simulink model "dead_time_generator"  (R2023b)
settings: Solver=VariableStepAuto  StartTime=0.0  StopTime=10.0  RelTol=1e-3
PreLoadFcn:
  | Fs = 10e4
  | Ts = 1/Fs
  | 
  | Tsamp = Ts/100;
  | 
  | Td = Tsamp*3
  | Zdelay = round(Td/Tsamp)
libraries: spsSawtoothGeneratorLib x1
settings Model: Creator=baik3-ad  LastModifiedBy=baik3-ad

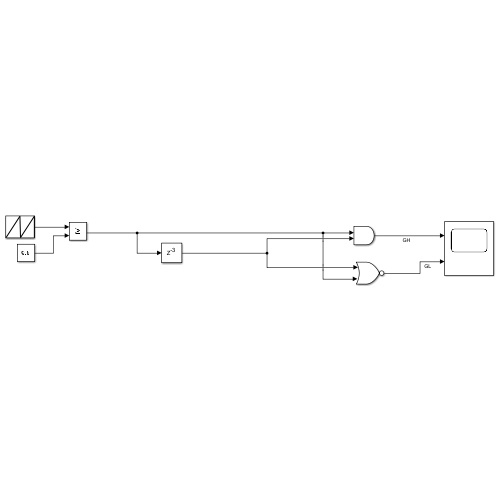
[thumbnail: Simulink's stored preview of the top-level diagram]
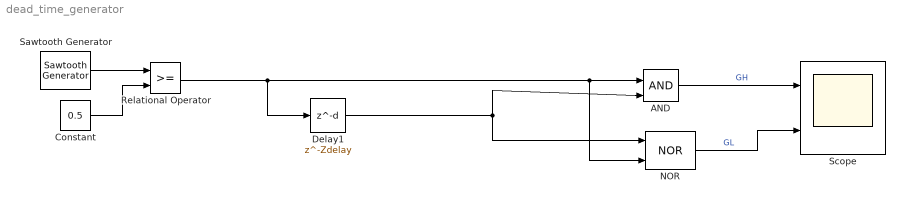
== system dead_time_generator ==
  AND : Logic  IconShape=distinctive  AllPortsSameDT=off  OutDataTypeStr=boolean
  Constant : Constant  Value=0.5
  Delay1 : Delay  DelayLength=Zdelay  InitialCondition=0
  NOR : Logic  Operator=NOR  IconShape=distinctive  AllPortsSameDT=off  OutDataTypeStr=boolean
  Relational Operator : RelationalOperator  OutDataTypeStr=boolean  RndMeth=Simplest  InputSameDT=off
  Sawtooth Generator : spsSawtoothGeneratorLib/Sawtooth Generator  Freq=Fs  Phase=0  Ts=Tsamp
  Scope : Scope  NumInputPorts=2
  wires:
  Sawtooth Generator/1 -> Relational Operator/1
  Constant/1 -> Relational Operator/2
  Relational Operator/1 -> Delay1/1, NOR/2, AND/1
  NOR/1 -> Scope/2  "GL"
  AND/1 -> Scope/1  "GH"
  Delay1/1 -> NOR/1, AND/2
